simulink model "Lab6_2017B5A30983P_Fullwave_Uncontrolled"  (R2019b)
settings: Solver=VariableStepAuto  StartTime=0.0  StopTime=0.06  RelTol=1e-3
libraries: powerlib x11, powerlib_meascontrol x2
settings Model: Creator=swaga  LastModifiedBy=swaga

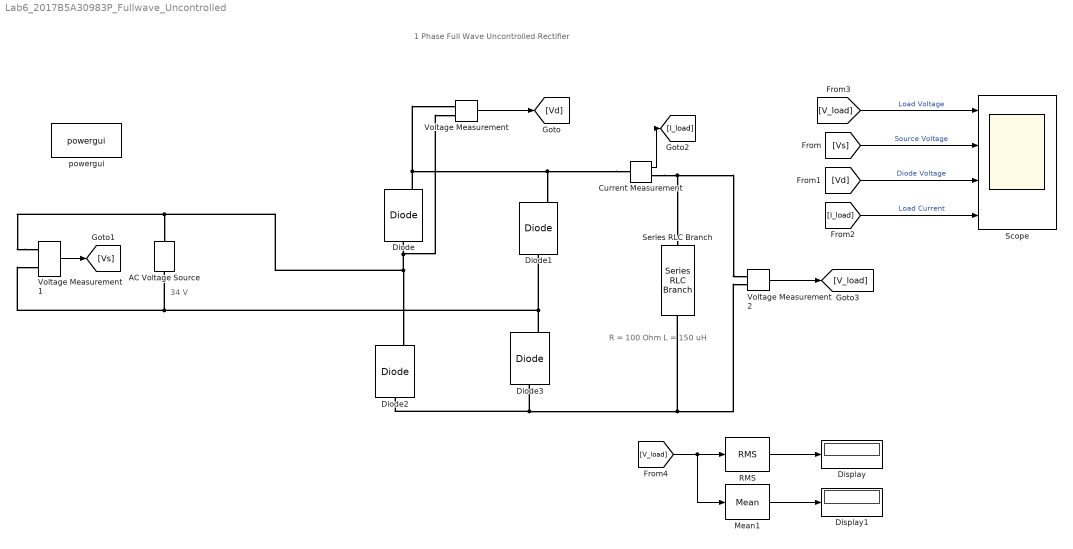
== system Lab6_2017B5A30983P_Fullwave_Uncontrolled ==
  note: 1 Phase Full Wave Uncontrolled Rectifier
  note: R = 100 Ohm
      | L =  150 uH
  note: 34 V
  AC Voltage Source : powerlib/Electrical Sources/AC Voltage Source  Amplitude=34  Phase=0  Frequency=50  SampleTime=0  Measurements=None  BusType=swing  Pref=10e3  Qref=0  Qmin=-inf  Qmax=+inf
      settings: SourceProductName=Simscape Electrical
  Current Measurement : powerlib/Measurements/Current Measurement  PhasorSimulation=off  OutputType=Complex  PSBequivalent=0
      settings: SourceProductName=Simscape Electrical
  Diode{,1..3} (4 alike) : powerlib/Power Electronics/Diode  Ron=0.001  Lon=0  Vf=0.8  IC=0  UseSnubber=0  Rs=500  Cs=250e-9  Measurements=on
      settings: SourceProductName=Simscape Electrical
  Display : Display
  Display1 : Display
  Mean1 : powerlib_meascontrol/Measurements/Mean  Freq=50  Vinit=0  Ts=0
      settings: SourceProductName=Simscape Electrical
  RMS : powerlib_meascontrol/Measurements/RMS  TrueRMS=on  Freq=50  RMSInit=120  Ts=0
      settings: SourceProductName=Simscape Electrical
  Scope : Scope  NumInputPorts=4
  Series RLC Branch : powerlib/Elements/Series RLC Branch  LConnTagsString=__new0  RConnTagsString=__new0  BranchType=R  Resistance=100  Inductance=150e-6  SetiL0=off  InitialCurrent=0  Capacitance=1e-6  Setx0=off  InitialVoltage=0  Measurements=None
      settings: SourceProductName=Simscape Electrical
  Voltage Measurement : powerlib/Measurements/Voltage Measurement  PhasorSimulation=off  OutputType=Complex  PSBequivalent=0
      settings: SourceProductName=Simscape Electrical
  Voltage Measurement1 : powerlib/Measurements/Voltage Measurement  PhasorSimulation=off  OutputType=Complex  PSBequivalent=0
      settings: SourceProductName=Simscape Electrical
  Voltage Measurement2 : powerlib/Measurements/Voltage Measurement  PhasorSimulation=off  OutputType=Complex  PSBequivalent=0
      settings: SourceProductName=Simscape Electrical
  powergui : powerlib/powergui  Priority=1  SimulationMode=Continuous  SampleTime=50e-6  frequency=60  Iterations=50  frequencyindice=50  Pbase=100e6  ErrMax=1e-4  UnitsV=kV  UnitsW=MW  buscounter=0  FunctionMessages=off  echomessages=off  EnableUseOfTLC=off  CurrentSourceSwitches=off  DisableSnubberDevices=off  DisableRonSwitches=off  DisableVfSwitches=off  DisplayEquations=off  AutomaticDiscreteSolvers=off  SolverType=Tustin/Backward Euler (TBE)  Interpol=off  ExternalGateDelay=off  methode=off  Ts=100  x0status=blocks  SPID=on  SwTol=0  HookPort=off  NonlinearTolerance=1e-4  nMaxIteration=100  ContinueOnMaxIteration=off  RestoreLinks=warning  ResistiveCurrentMeasurement=off  Frange=[0:2:500]  Ylog=off  Xlog=on  ShowGrid=off  save=off  variable=ZData  structure=0  ZoomFFT=off  StartTime=0.0  cycles=1  DisplayStyle=1  fundamental=60  FreqAxis=off  MaxFrequency=1000  frequencyindicesteady=1  RmsSteady=1  display=off
      settings: SourceProductName=Simscape Electrical
  wires:
  Voltage Measurement1/1 -> [Vs]
  [Vd] -> Scope/3  "Diode Voltage"
  Voltage Measurement2/1 -> [V_load]
  [V_load] -> Mean1/1, RMS/1
  [Vs] -> Scope/2  "Source Voltage"
  RMS/1 -> Display/1
  Current Measurement/1 -> [I_load]
  Mean1/1 -> Display1/1
  [V_load] -> Scope/1  "Load Voltage"
  [I_load] -> Scope/4  "Load Current"
  Voltage Measurement/1 -> [Vd]
  connections:
  Voltage Measurement1/LConn1 -- AC Voltage Source/RConn1 -- Diode2/RConn1 -- Voltage Measurement/LConn2 -- Diode/LConn1
  AC Voltage Source/LConn1 -- Diode3/RConn1 -- Diode1/LConn1 -- Voltage Measurement1/LConn2
  Series RLC Branch/RConn1 -- Diode2/LConn1 -- Diode3/LConn1 -- Voltage Measurement2/LConn2
  Voltage Measurement2/LConn1 -- Series RLC Branch/LConn1 -- Current Measurement/RConn1
  Current Measurement/LConn1 -- Voltage Measurement/LConn1 -- Diode/RConn1 -- Diode1/RConn1
